simulink model "Project_B_Simulink_Model"  (R2019b)
settings: Solver=VariableStepAuto  StartTime=0.0  StopTime=2  RelTol=1e-3
undefined symbols (not defined in the file or in its folder): Fs
libraries: dspfdesign x1
settings Model: Creator=kerem  LastModifiedBy=kerem

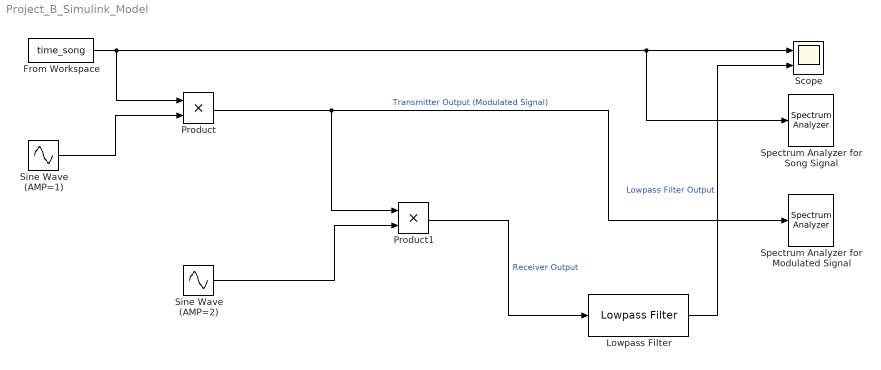
== system Project_B_Simulink_Model ==
  From Workspace : FromWorkspace  VariableName=time_song  OutDataTypeStr=double  SampleTime=1/Fs  Interpolate=off  OutputAfterFinalValue=Setting to zero
  Lowpass Filter : dspfdesign/Lowpass Filter  FilterType=FIR  DesignForMinimumOrder=on  FilterOrder=50  PassbandFrequency=25e3  StopbandFrequency=30e3  PassbandRipple=0.1  StopbandAttenuation=80  InheritSampleRate=off  SampleRate=Fs  SimulateUsing=Code generation  roundingMode=Floor  coeffsDataTypeStr=fixdt(1,16)
  Product : Product
  Product1 : Product
  Scope : Scope  NumInputPorts=2
  "Sine Wave (AMP=1) " : Sin  Frequency=60e3*2*pi  SampleTime=1/Fs
  Sine Wave (AMP=2) : Sin  Amplitude=2  Frequency=60e3*2*pi  SampleTime=1/Fs
  Spectrum Analyzer for Modulated Signal : SpectrumAnalyzer
  Spectrum Analyzer for Song Signal : SpectrumAnalyzer
  wires:
  From Workspace/1 -> Product/1, Spectrum Analyzer for Song Signal/1, Scope/1
  "Sine Wave (AMP=1) "/1 -> Product/2
  Product/1 -> Product1/1, Spectrum Analyzer for Modulated Signal/1  "Transmitter Output (Modulated Signal)"
  Sine Wave (AMP=2)/1 -> Product1/2
  Product1/1 -> Lowpass Filter/1  "Receiver Output"
  Lowpass Filter/1 -> Scope/2  "Lowpass Filter Output"
